simulink model "pulse"  (R2015a)
settings: Solver=ode45  StartTime=0.0  StopTime=10.0  RelTol=1e-3
libraries: simulink x1
settings Model: Creator=dhairya  LastModifiedBy=dhairya

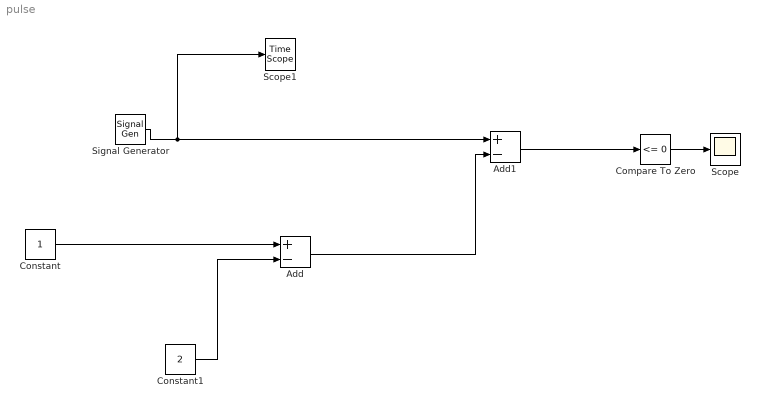
== system pulse ==
  Add : Sum  Inputs=+-
  Add1 : Sum  Inputs=+-
  Compare To Zero : simulink/Logic and Bit Operations/Compare To Zero  relop=<=  OutDataTypeStr=boolean
  Constant : Constant
  Constant1 : Constant  Value=2
  Scope : Scope
  Scope1 : TimeScope
  Signal Generator : SignalGenerator  Amplitude=5  Frequency=10
  wires:
  Constant/1 -> Add/1
  Constant1/1 -> Add/2
  Signal Generator/1 -> Scope1/1, Add1/1
  Add/1 -> Add1/2
  Add1/1 -> Compare To Zero/1
  Compare To Zero/1 -> Scope/1
